simulink model "untitled2"  (R2022b)
settings: Solver=VariableStepAuto  StartTime=0.0  StopTime=10.0  RelTol=1e-3
settings Model: Creator=admin  LastModifiedBy=admin

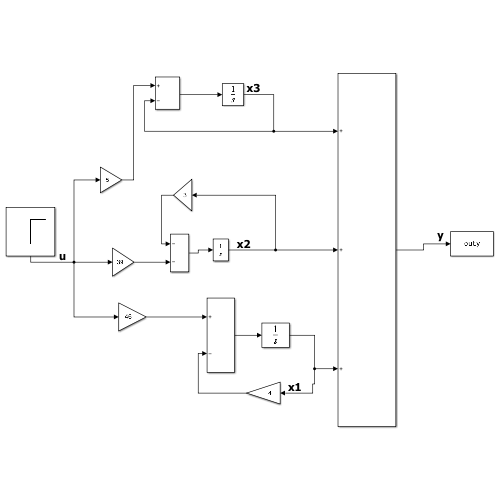
[thumbnail: Simulink's stored preview of the top-level diagram]
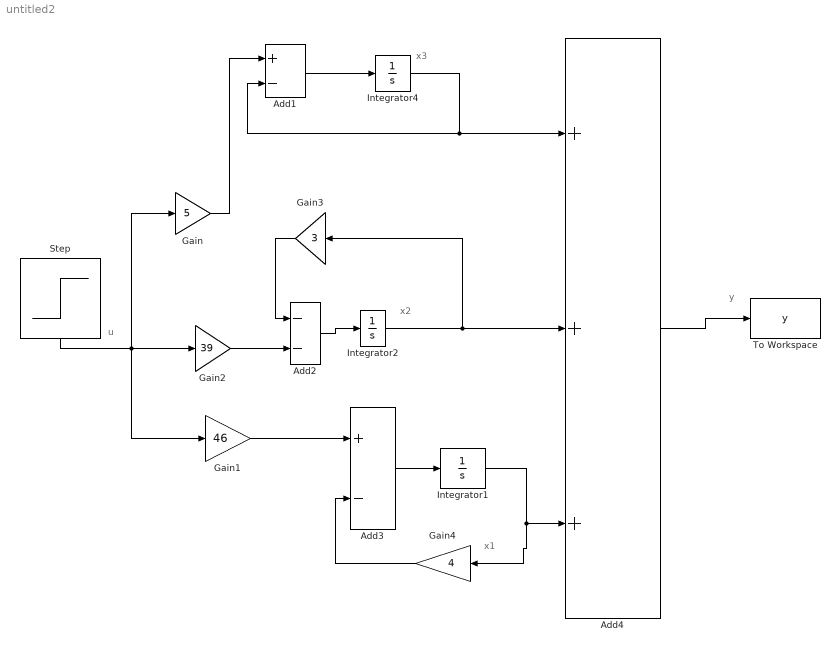
== system untitled2 ==
  note: x3
  note: x2
  note: x1
  note: y
  note: u
  Add1 : Sum  Inputs=+-
  Add2 : Sum  Inputs=--
  Add3 : Sum  Inputs=+-
  Add4 : Sum  Inputs=+++
  Gain : Gain  Gain=5
  Gain1 : Gain  Gain=46
  Gain2 : Gain  Gain=39
  Gain3 : Gain  Gain=3
  Gain4 : Gain  Gain=4
  Integrator1 : Integrator
  Integrator2 : Integrator
  Integrator4 : Integrator
  Step : Step  SampleTime=0
  To Workspace : ToWorkspace  VariableName=y  SaveFormat=Structure With Time  SampleTime=-1
  wires:
  Step/1 -> Gain/1, Gain2/1, Gain1/1
  Gain2/1 -> Add2/2
  Gain/1 -> Add1/1
  Gain1/1 -> Add3/1
  Gain4/1 -> Add3/2
  Add3/1 -> Integrator1/1
  Integrator1/1 -> Gain4/1, Add4/3
  Gain3/1 -> Add2/1
  Add2/1 -> Integrator2/1
  Integrator2/1 -> Gain3/1, Add4/2
  Add1/1 -> Integrator4/1
  Integrator4/1 -> Add1/2, Add4/1
  Add4/1 -> To Workspace/1
